simulink model "P5OscarAvila"  (R2018a)
settings: Solver=VariableStepAuto  StartTime=0.0  StopTime=60  FixedStep=0.02  RelTol=1e-3
settings Model: Creator=Oscar  LastModifiedBy=Oscar

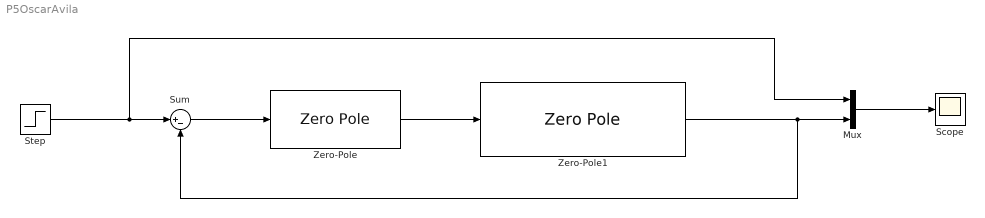
== system P5OscarAvila ==
  Mux : Mux  Inputs=2
  Scope : Scope
  Step : Step  SampleTime=0
  Sum : Sum  Inputs=|+-
  Zero-Pole : ZeroPole  Zeros=[0.916]  Poles=[3.537]  Gain=2.0002
  Zero-Pole1 : ZeroPole  Zeros=[-2729 100]  Poles=[-1 -9.967]  Gain=-3.6519e-05
  wires:
  Zero-Pole1/1 -> Sum/2, Mux/2
  Sum/1 -> Zero-Pole/1
  Step/1 -> Mux/1, Sum/1
  Zero-Pole/1 -> Zero-Pole1/1
  Mux/1 -> Scope/1
